simulink model "Input_Model"  (R2016b)
settings: Solver=VariableStepAuto  StartTime=0.0  StopTime=inf  RelTol=1e-3
libraries: vrlib x1
settings Model: Creator=Dylan  LastModifiedBy=Dylan

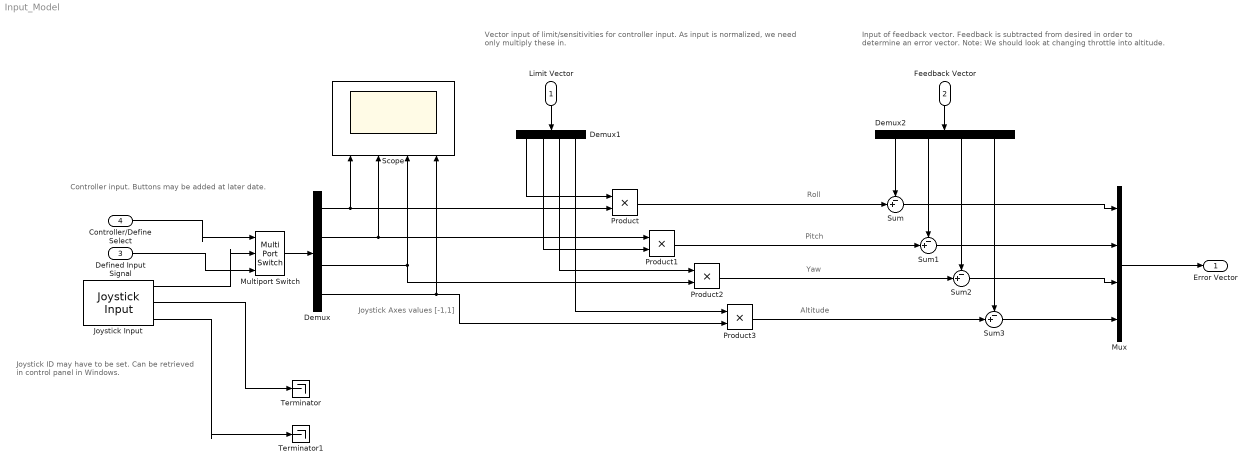
== system Input_Model ==
  note: Input of feedback vector.  Feedback is subtracted from desired
      | in order to determine an error vector.
      | Note: We should look at changing throttle into altitude.
  note: Vector input of limit/sensitivities for controller input.  As input is
      | normalized, we need only multiply these in.
  note: Controller input.
      | Buttons may be added at later date.
  note: Altitude
  note: Yaw
  note: Pitch
  note: Roll
  note: Joystick Axes values [-1,1]
  note: Joystick ID may have to be set.
      | Can be retrieved in control panel in Windows.
  Limit Vector : Inport  PortDimensions=4
  Feedback Vector : Inport  Port=2  PortDimensions=4
  Defined Input Signal : Inport  Port=3  PortDimensions=4
  Controller/Define Select : Inport  Port=4
  Demux : Demux
  Demux1 : Demux
  Demux2 : Demux
  Joystick Input : vrlib/Joystick Input  joyid=0  adjustports=on  forcefeed=off
  Multiport Switch : MultiPortSwitch  DataPortOrder=Zero-based contiguous  Inputs=2
  Mux : Mux
  Product{,1..3} (4 alike) : Product
  Scope : Scope  NumInputPorts=4
  Sum{,1..3} (4 alike) : Sum  Inputs=-+|
  Terminator : Terminator
  Terminator1 : Terminator
  Error Vector : Outport
  wires:
  Demux/4 -> Product3/2, Scope/4
  Demux/3 -> Scope/3, Product2/2
  Demux/2 -> Product1/1, Scope/2
  Demux/1 -> Scope/1, Product/2
  Joystick Input/2 -> Terminator/1
  Limit Vector/1 -> Demux1/1
  Demux1/1 -> Product/1
  Demux1/2 -> Product1/2
  Demux1/3 -> Product2/1
  Demux1/4 -> Product3/1
  Feedback Vector/1 -> Demux2/1
  Product/1 -> Sum/2
  Demux2/1 -> Sum/1
  Demux2/2 -> Sum1/1
  Product1/1 -> Sum1/2
  Demux2/3 -> Sum2/1
  Product2/1 -> Sum2/2
  Product3/1 -> Sum3/2
  Demux2/4 -> Sum3/1
  Sum2/1 -> Mux/3
  Sum1/1 -> Mux/2
  Sum/1 -> Mux/1
  Sum3/1 -> Mux/4
  Mux/1 -> Error Vector/1
  Controller/Define Select/1 -> Multiport Switch/1
  Multiport Switch/1 -> Demux/1
  Defined Input Signal/1 -> Multiport Switch/3
  Joystick Input/1 -> Multiport Switch/2
  Joystick Input/3 -> Terminator1/1
